simulink library "LibDBC_SCU_ch1"  (R2024b)
settings: Solver=VariableStepAuto  StartTime=0.0  StopTime=10.0  RelTol=1e-3
undefined symbols (not defined in the file): bit_packing, bit_unpacking, IO_Blk_Lib_TTC500, IO_CAN_ConfigMsg, IO_CAN_ReadMsg
libraries: simulink x59, IOBlock_Library_TTC580 x32
(part 15 of 21)

== system LibDBC_SCU_ch1/mBMS_PP ==
  note: Don't change the Names of the Blocks
  IO_CAN_ConfigMsg : Subsystem  mask(IO_CAN_ConfigMsg_Code){SampleTime=-1, ttlib=IO_Blk_Lib_TTC500, ttDescription=IO_CAN_ConfigMsg, tt_iolib_version=0.19, channel=IO_CAN_CHANNEL_1, mode=IO_CAN_MSG_READ, id_format=IO_CAN_STD_FRAME, id=0x112, ac_mask=0x7FF}
      mask help: Configures a message object for the given CAN channel.
      mask init:
      | %
      mask Help: web(which('IO_CAN.h'))
      mask TypeOptions channel: IO_CAN_CHANNEL_0  | IO_CAN_CHANNEL_1 | IO_CAN_CHANNEL_2 | IO_CAN_CHANNEL_3 | IO_CAN_CHANNEL_4 | IO_CAN_CHANNEL_5 | IO_CAN_CHANNEL_6
      mask Callback channel: %
      mask TypeOptions mode: IO_CAN_MSG_READ | IO_CAN_MSG_WRITE
      mask Callback mode: %
      mask TypeOptions id_format: IO_CAN_STD_FRAME | IO_CAN_EXT_FRAME
      mask Callback id_format: %
      mask Callback id: %
      mask Callback ac_mask: %
  IO_CAN_ReadMsg : Subsystem  mask(IO_CAN_ReadMsg_Code){SampleTime=-1, ttlib=IO_Blk_Lib_TTC500, ttDescription=IO_CAN_ReadMsg, tt_iolib_version=0.19}
      mask help: Reads a message from a given message object.
      mask init:
      | %
      mask Help: web(which('IO_CAN.h'))
  Terminator{2,6..8} (4 alike) : Terminator
  Trigger_Block : Subsystem  mask(Derate Trigger){derate=10, trigger_offset=0}
      mask prompts: trigger_offset "offset for the trigger"
      mask help: derate "n": every n-th cylce a trigger is submitted
  bit_unpacking1 : Subsystem  LoadFcn=|  mask(bit_unpacking_Code){SampleTime=-1, ttlib=IO_Blk_Lib_TTC500, ttDescription=bit_unpacking, tt_iolib_version=0.26, Endianness=little, Format=unsigned, Inversion=off, Startbit=0, Width_bits=16, Factor=0.1, Offset=0}
      | try
      | %
      | %Upgrade Information - standard BEGIN
      | new_color = 'blue';
      | new_ver = '0.26';
      | act_ver = get_param(gcb,'tt_iolib_version');
      | if not(strcmp(act_ver,new_ver))
      |     disp(['Upgrade block: ',gcb,char(10),'       Version: ',act_ver,' to ',new_ver]);
      |     %switch - case for specific upgrade information e.g. additional parameter required 
      |     %Change appearance and version information
      |     set_param(gcb,'ForegroundColor',new_color);
      |     set_param(gcb,'tt_iolib_version',new_ver);
      | end
      | %Upgrade Information - standard END
      | catch
      | %Standard catch section BEGIN
      | errordlg('An error occurred in a callback of the TTC580-BlockLib. Please open the Diagnostic Viewer for further details');
      | disp(' ');
      | disp('------------------------------------------------------------');
      | disp('An error occurred in a callback of the TTC580-BlockLib.');
      | disp(['Please check the parameters in the mask of ',gcb]);
      | disp('If you do not encounter any violations, then please '); 
      | disp('copy the following lines and report this to support@ttcontrol.com ');
      | disp('<< begin of error message dump >>');
      | disp(['Version of TTC580-BlockLib: ', get_param(gcb,'tt_iolib_version')]);
      | disp(get_param(gcb,'ttDescription'));
      | disp(gcb);
      | x=lasterror;disp(x.message);
      | disp(get_param(gcb,'MaskValues'));
      | disp(version);
      | disp(computer);
      | disp('<< end of error message dump >>');
      | disp('------------------------------------------------------------');
      | disp(' ');
      | %Standard catch section END
      | end
      mask help:
      | Block to read in CAN signal from a specified position within 64bit field.
      | For "Factor" and "Offset" the definition of Vector's CANdb applies:
      | [Physical value] = ( [Raw value] * [Factor] ) + [Offset]
      | with Raw value of a signal being the value as it is transmitted in the CAN-network
      | Verification capabilities are supported.
      mask init: same as LibDBC_SCU_ch1/EXT_BalancingRequest/bit_packing1
      mask Help: web([which('usermanual.html'),'#',lower(get_param(gcb,'ttDescription'))])
      mask TypeOptions Endianness: big | little
      mask Callback Endianness: %
      mask TypeOptions Format: unsigned | signed | real32
      mask Callback Format: %
      mask Callback Inversion: %
      mask Callback Startbit: %
      mask Callback Width_bits: %
      mask Callback Factor: %
      mask Callback Offset: %
  bit_unpacking2 : Subsystem  LoadFcn=|  mask(bit_unpacking_Code){SampleTime=-1, ttlib=IO_Blk_Lib_TTC500, ttDescription=bit_unpacking, tt_iolib_version=0.26, Endianness=little, Format=unsigned, Inversion=off, Startbit=16, Width_bits=16, Factor=1, Offset=0}
      | try
      | %
      | %Upgrade Information - standard BEGIN
      | new_color = 'blue';
      | new_ver = '0.26';
      | act_ver = get_param(gcb,'tt_iolib_version');
      | if not(strcmp(act_ver,new_ver))
      |     disp(['Upgrade block: ',gcb,char(10),'       Version: ',act_ver,' to ',new_ver]);
      |     %switch - case for specific upgrade information e.g. additional parameter required 
      |     %Change appearance and version information
      |     set_param(gcb,'ForegroundColor',new_color);
      |     set_param(gcb,'tt_iolib_version',new_ver);
      | end
      | %Upgrade Information - standard END
      | catch
      | %Standard catch section BEGIN
      | errordlg('An error occurred in a callback of the TTC580-BlockLib. Please open the Diagnostic Viewer for further details');
      | disp(' ');
      | disp('------------------------------------------------------------');
      | disp('An error occurred in a callback of the TTC580-BlockLib.');
      | disp(['Please check the parameters in the mask of ',gcb]);
      | disp('If you do not encounter any violations, then please '); 
      | disp('copy the following lines and report this to support@ttcontrol.com ');
      | disp('<< begin of error message dump >>');
      | disp(['Version of TTC580-BlockLib: ', get_param(gcb,'tt_iolib_version')]);
      | disp(get_param(gcb,'ttDescription'));
      | disp(gcb);
      | x=lasterror;disp(x.message);
      | disp(get_param(gcb,'MaskValues'));
      | disp(version);
      | disp(computer);
      | disp('<< end of error message dump >>');
      | disp('------------------------------------------------------------');
      | disp(' ');
      | %Standard catch section END
      | end
      mask help:
      | Block to read in CAN signal from a specified position within 64bit field.
      | For "Factor" and "Offset" the definition of Vector's CANdb applies:
      | [Physical value] = ( [Raw value] * [Factor] ) + [Offset]
      | with Raw value of a signal being the value as it is transmitted in the CAN-network
      | Verification capabilities are supported.
      mask init: same as LibDBC_SCU_ch1/EXT_BalancingRequest/bit_packing1
      mask Help: web([which('usermanual.html'),'#',lower(get_param(gcb,'ttDescription'))])
      mask TypeOptions Endianness: big | little
      mask Callback Endianness: %
      mask TypeOptions Format: unsigned | signed | real32
      mask Callback Format: %
      mask Callback Inversion: %
      mask Callback Startbit: %
      mask Callback Width_bits: %
      mask Callback Factor: %
      mask Callback Offset: %
  bit_unpacking3 : Subsystem  LoadFcn=|  mask(bit_unpacking_Code){SampleTime=-1, ttlib=IO_Blk_Lib_TTC500, ttDescription=bit_unpacking, tt_iolib_version=0.26, Endianness=little, Format=unsigned, Inversion=off, Startbit=32, Width_bits=16, Factor=0.1, Offset=0}
      | try
      | %
      | %Upgrade Information - standard BEGIN
      | new_color = 'blue';
      | new_ver = '0.26';
      | act_ver = get_param(gcb,'tt_iolib_version');
      | if not(strcmp(act_ver,new_ver))
      |     disp(['Upgrade block: ',gcb,char(10),'       Version: ',act_ver,' to ',new_ver]);
      |     %switch - case for specific upgrade information e.g. additional parameter required 
      |     %Change appearance and version information
      |     set_param(gcb,'ForegroundColor',new_color);
      |     set_param(gcb,'tt_iolib_version',new_ver);
      | end
      | %Upgrade Information - standard END
      | catch
      | %Standard catch section BEGIN
      | errordlg('An error occurred in a callback of the TTC580-BlockLib. Please open the Diagnostic Viewer for further details');
      | disp(' ');
      | disp('------------------------------------------------------------');
      | disp('An error occurred in a callback of the TTC580-BlockLib.');
      | disp(['Please check the parameters in the mask of ',gcb]);
      | disp('If you do not encounter any violations, then please '); 
      | disp('copy the following lines and report this to support@ttcontrol.com ');
      | disp('<< begin of error message dump >>');
      | disp(['Version of TTC580-BlockLib: ', get_param(gcb,'tt_iolib_version')]);
      | disp(get_param(gcb,'ttDescription'));
      | disp(gcb);
      | x=lasterror;disp(x.message);
      | disp(get_param(gcb,'MaskValues'));
      | disp(version);
      | disp(computer);
      | disp('<< end of error message dump >>');
      | disp('------------------------------------------------------------');
      | disp(' ');
      | %Standard catch section END
      | end
      mask help:
      | Block to read in CAN signal from a specified position within 64bit field.
      | For "Factor" and "Offset" the definition of Vector's CANdb applies:
      | [Physical value] = ( [Raw value] * [Factor] ) + [Offset]
      | with Raw value of a signal being the value as it is transmitted in the CAN-network
      | Verification capabilities are supported.
      mask init: same as LibDBC_SCU_ch1/EXT_BalancingRequest/bit_packing1
      mask Help: web([which('usermanual.html'),'#',lower(get_param(gcb,'ttDescription'))])
      mask TypeOptions Endianness: big | little
      mask Callback Endianness: %
      mask TypeOptions Format: unsigned | signed | real32
      mask Callback Format: %
      mask Callback Inversion: %
      mask Callback Startbit: %
      mask Callback Width_bits: %
      mask Callback Factor: %
      mask Callback Offset: %
  bit_unpacking4 : Subsystem  LoadFcn=|  mask(bit_unpacking_Code){SampleTime=-1, ttlib=IO_Blk_Lib_TTC500, ttDescription=bit_unpacking, tt_iolib_version=0.26, Endianness=little, Format=unsigned, Inversion=off, Startbit=48, Width_bits=16, Factor=1, Offset=0}
      | try
      | %
      | %Upgrade Information - standard BEGIN
      | new_color = 'blue';
      | new_ver = '0.26';
      | act_ver = get_param(gcb,'tt_iolib_version');
      | if not(strcmp(act_ver,new_ver))
      |     disp(['Upgrade block: ',gcb,char(10),'       Version: ',act_ver,' to ',new_ver]);
      |     %switch - case for specific upgrade information e.g. additional parameter required 
      |     %Change appearance and version information
      |     set_param(gcb,'ForegroundColor',new_color);
      |     set_param(gcb,'tt_iolib_version',new_ver);
      | end
      | %Upgrade Information - standard END
      | catch
      | %Standard catch section BEGIN
      | errordlg('An error occurred in a callback of the TTC580-BlockLib. Please open the Diagnostic Viewer for further details');
      | disp(' ');
      | disp('------------------------------------------------------------');
      | disp('An error occurred in a callback of the TTC580-BlockLib.');
      | disp(['Please check the parameters in the mask of ',gcb]);
      | disp('If you do not encounter any violations, then please '); 
      | disp('copy the following lines and report this to support@ttcontrol.com ');
      | disp('<< begin of error message dump >>');
      | disp(['Version of TTC580-BlockLib: ', get_param(gcb,'tt_iolib_version')]);
      | disp(get_param(gcb,'ttDescription'));
      | disp(gcb);
      | x=lasterror;disp(x.message);
      | disp(get_param(gcb,'MaskValues'));
      | disp(version);
      | disp(computer);
      | disp('<< end of error message dump >>');
      | disp('------------------------------------------------------------');
      | disp(' ');
      | %Standard catch section END
      | end
      mask help:
      | Block to read in CAN signal from a specified position within 64bit field.
      | For "Factor" and "Offset" the definition of Vector's CANdb applies:
      | [Physical value] = ( [Raw value] * [Factor] ) + [Offset]
      | with Raw value of a signal being the value as it is transmitted in the CAN-network
      | Verification capabilities are supported.
      mask init: same as LibDBC_SCU_ch1/EXT_BalancingRequest/bit_packing1
      mask Help: web([which('usermanual.html'),'#',lower(get_param(gcb,'ttDescription'))])
      mask TypeOptions Endianness: big | little
      mask Callback Endianness: %
      mask TypeOptions Format: unsigned | signed | real32
      mask Callback Format: %
      mask Callback Inversion: %
      mask Callback Startbit: %
      mask Callback Width_bits: %
      mask Callback Factor: %
      mask Callback Offset: %
  PP_I_chrg : Outport  VectorParamsAs1DForOutWhenUnconnected=off
  PP_Pwr_chrg : Outport  Port=2  VectorParamsAs1DForOutWhenUnconnected=off
  PP_I_dschrg : Outport  Port=3  VectorParamsAs1DForOutWhenUnconnected=off
  PP_Pwr_dschrg : Outport  Port=4  VectorParamsAs1DForOutWhenUnconnected=off
  ErrorCode : Outport  Port=5  VectorParamsAs1DForOutWhenUnconnected=off
  wires:
  IO_CAN_ReadMsg/3(buffer_length) -> Terminator8/1
  IO_CAN_ReadMsg/4(buffer_id_format) -> Terminator7/1
  IO_CAN_ReadMsg/5(buffer_id) -> Terminator6/1
  IO_CAN_ConfigMsg/2(handle) -> IO_CAN_ReadMsg/1(handle)
  IO_CAN_ConfigMsg/1(ErrorCode) -> Terminator2/1
  Trigger_Block/1(Trigger) -> IO_CAN_ReadMsg/Enable
  IO_CAN_ReadMsg/1(ErrorCode) -> ErrorCode/1
  IO_CAN_ReadMsg/2(buffer_data) -> bit_unpacking1/1(Data_in), bit_unpacking2/1(Data_in), bit_unpacking3/1(Data_in), bit_unpacking4/1(Data_in)
  bit_unpacking1/1(Data_out) -> PP_I_chrg/1
  bit_unpacking2/1(Data_out) -> PP_Pwr_chrg/1
  bit_unpacking3/1(Data_out) -> PP_I_dschrg/1
  bit_unpacking4/1(Data_out) -> PP_Pwr_dschrg/1

== system LibDBC_SCU_ch1/mBMS_RI_OCV_Approx ==
  note: Don't change the Names of the Blocks
  IO_CAN_ConfigMsg : Subsystem  mask(IO_CAN_ConfigMsg_Code){SampleTime=-1, ttlib=IO_Blk_Lib_TTC500, ttDescription=IO_CAN_ConfigMsg, tt_iolib_version=0.19, channel=IO_CAN_CHANNEL_1, mode=IO_CAN_MSG_READ, id_format=IO_CAN_STD_FRAME, id=0x113, ac_mask=0x7FF}
      mask help: Configures a message object for the given CAN channel.
      mask init:
      | %
      mask Help: web(which('IO_CAN.h'))
      mask TypeOptions channel: IO_CAN_CHANNEL_0  | IO_CAN_CHANNEL_1 | IO_CAN_CHANNEL_2 | IO_CAN_CHANNEL_3 | IO_CAN_CHANNEL_4 | IO_CAN_CHANNEL_5 | IO_CAN_CHANNEL_6
      mask Callback channel: %
      mask TypeOptions mode: IO_CAN_MSG_READ | IO_CAN_MSG_WRITE
      mask Callback mode: %
      mask TypeOptions id_format: IO_CAN_STD_FRAME | IO_CAN_EXT_FRAME
      mask Callback id_format: %
      mask Callback id: %
      mask Callback ac_mask: %
  IO_CAN_ReadMsg : Subsystem  mask(IO_CAN_ReadMsg_Code){SampleTime=-1, ttlib=IO_Blk_Lib_TTC500, ttDescription=IO_CAN_ReadMsg, tt_iolib_version=0.19}
      mask help: Reads a message from a given message object.
      mask init:
      | %
      mask Help: web(which('IO_CAN.h'))
  Terminator{2,6..8} (4 alike) : Terminator
  Trigger_Block : Subsystem  mask(Derate Trigger){derate=10, trigger_offset=0}
      mask prompts: trigger_offset "offset for the trigger"
      mask help: derate "n": every n-th cylce a trigger is submitted
  bit_unpacking1 : Subsystem  LoadFcn=|  mask(bit_unpacking_Code){SampleTime=-1, ttlib=IO_Blk_Lib_TTC500, ttDescription=bit_unpacking, tt_iolib_version=0.26, Endianness=little, Format=unsigned, Inversion=off, Startbit=0, Width_bits=16, Factor=0.01, Offset=0}
      | try
      | %
      | %Upgrade Information - standard BEGIN
      | new_color = 'blue';
      | new_ver = '0.26';
      | act_ver = get_param(gcb,'tt_iolib_version');
      | if not(strcmp(act_ver,new_ver))
      |     disp(['Upgrade block: ',gcb,char(10),'       Version: ',act_ver,' to ',new_ver]);
      |     %switch - case for specific upgrade information e.g. additional parameter required 
      |     %Change appearance and version information
      |     set_param(gcb,'ForegroundColor',new_color);
      |     set_param(gcb,'tt_iolib_version',new_ver);
      | end
      | %Upgrade Information - standard END
      | catch
      | %Standard catch section BEGIN
      | errordlg('An error occurred in a callback of the TTC580-BlockLib. Please open the Diagnostic Viewer for further details');
      | disp(' ');
      | disp('------------------------------------------------------------');
      | disp('An error occurred in a callback of the TTC580-BlockLib.');
      | disp(['Please check the parameters in the mask of ',gcb]);
      | disp('If you do not encounter any violations, then please '); 
      | disp('copy the following lines and report this to support@ttcontrol.com ');
      | disp('<< begin of error message dump >>');
      | disp(['Version of TTC580-BlockLib: ', get_param(gcb,'tt_iolib_version')]);
      | disp(get_param(gcb,'ttDescription'));
      | disp(gcb);
      | x=lasterror;disp(x.message);
      | disp(get_param(gcb,'MaskValues'));
      | disp(version);
      | disp(computer);
      | disp('<< end of error message dump >>');
      | disp('------------------------------------------------------------');
      | disp(' ');
      | %Standard catch section END
      | end
      mask help:
      | Block to read in CAN signal from a specified position within 64bit field.
      | For "Factor" and "Offset" the definition of Vector's CANdb applies:
      | [Physical value] = ( [Raw value] * [Factor] ) + [Offset]
      | with Raw value of a signal being the value as it is transmitted in the CAN-network
      | Verification capabilities are supported.
      mask init: same as LibDBC_SCU_ch1/EXT_BalancingRequest/bit_packing1
      mask Help: web([which('usermanual.html'),'#',lower(get_param(gcb,'ttDescription'))])
      mask TypeOptions Endianness: big | little
      mask Callback Endianness: %
      mask TypeOptions Format: unsigned | signed | real32
      mask Callback Format: %
      mask Callback Inversion: %
      mask Callback Startbit: %
      mask Callback Width_bits: %
      mask Callback Factor: %
      mask Callback Offset: %
  bit_unpacking2 : Subsystem  LoadFcn=|  mask(bit_unpacking_Code){SampleTime=-1, ttlib=IO_Blk_Lib_TTC500, ttDescription=bit_unpacking, tt_iolib_version=0.26, Endianness=little, Format=unsigned, Inversion=off, Startbit=16, Width_bits=16, Factor=0.01, Offset=0}
      | try
      | %
      | %Upgrade Information - standard BEGIN
      | new_color = 'blue';
      | new_ver = '0.26';
      | act_ver = get_param(gcb,'tt_iolib_version');
      | if not(strcmp(act_ver,new_ver))
      |     disp(['Upgrade block: ',gcb,char(10),'       Version: ',act_ver,' to ',new_ver]);
      |     %switch - case for specific upgrade information e.g. additional parameter required 
      |     %Change appearance and version information
      |     set_param(gcb,'ForegroundColor',new_color);
      |     set_param(gcb,'tt_iolib_version',new_ver);
      | end
      | %Upgrade Information - standard END
      | catch
      | %Standard catch section BEGIN
      | errordlg('An error occurred in a callback of the TTC580-BlockLib. Please open the Diagnostic Viewer for further details');
      | disp(' ');
      | disp('------------------------------------------------------------');
      | disp('An error occurred in a callback of the TTC580-BlockLib.');
      | disp(['Please check the parameters in the mask of ',gcb]);
      | disp('If you do not encounter any violations, then please '); 
      | disp('copy the following lines and report this to support@ttcontrol.com ');
      | disp('<< begin of error message dump >>');
      | disp(['Version of TTC580-BlockLib: ', get_param(gcb,'tt_iolib_version')]);
      | disp(get_param(gcb,'ttDescription'));
      | disp(gcb);
      | x=lasterror;disp(x.message);
      | disp(get_param(gcb,'MaskValues'));
      | disp(version);
      | disp(computer);
      | disp('<< end of error message dump >>');
      | disp('------------------------------------------------------------');
      | disp(' ');
      | %Standard catch section END
      | end
      mask help:
      | Block to read in CAN signal from a specified position within 64bit field.
      | For "Factor" and "Offset" the definition of Vector's CANdb applies:
      | [Physical value] = ( [Raw value] * [Factor] ) + [Offset]
      | with Raw value of a signal being the value as it is transmitted in the CAN-network
      | Verification capabilities are supported.
      mask init: same as LibDBC_SCU_ch1/EXT_BalancingRequest/bit_packing1
      mask Help: web([which('usermanual.html'),'#',lower(get_param(gcb,'ttDescription'))])
      mask TypeOptions Endianness: big | little
      mask Callback Endianness: %
      mask TypeOptions Format: unsigned | signed | real32
      mask Callback Format: %
      mask Callback Inversion: %
      mask Callback Startbit: %
      mask Callback Width_bits: %
      mask Callback Factor: %
      mask Callback Offset: %
  bit_unpacking3 : Subsystem  LoadFcn=|  mask(bit_unpacking_Code){SampleTime=-1, ttlib=IO_Blk_Lib_TTC500, ttDescription=bit_unpacking, tt_iolib_version=0.26, Endianness=little, Format=unsigned, Inversion=off, Startbit=32, Width_bits=16, Factor=0.01, Offset=0}
      | try
      | %
      | %Upgrade Information - standard BEGIN
      | new_color = 'blue';
      | new_ver = '0.26';
      | act_ver = get_param(gcb,'tt_iolib_version');
      | if not(strcmp(act_ver,new_ver))
      |     disp(['Upgrade block: ',gcb,char(10),'       Version: ',act_ver,' to ',new_ver]);
      |     %switch - case for specific upgrade information e.g. additional parameter required 
      |     %Change appearance and version information
      |     set_param(gcb,'ForegroundColor',new_color);
      |     set_param(gcb,'tt_iolib_version',new_ver);
      | end
      | %Upgrade Information - standard END
      | catch
      | %Standard catch section BEGIN
      | errordlg('An error occurred in a callback of the TTC580-BlockLib. Please open the Diagnostic Viewer for further details');
      | disp(' ');
      | disp('------------------------------------------------------------');
      | disp('An error occurred in a callback of the TTC580-BlockLib.');
      | disp(['Please check the parameters in the mask of ',gcb]);
      | disp('If you do not encounter any violations, then please '); 
      | disp('copy the following lines and report this to support@ttcontrol.com ');
      | disp('<< begin of error message dump >>');
      | disp(['Version of TTC580-BlockLib: ', get_param(gcb,'tt_iolib_version')]);
      | disp(get_param(gcb,'ttDescription'));
      | disp(gcb);
      | x=lasterror;disp(x.message);
      | disp(get_param(gcb,'MaskValues'));
      | disp(version);
      | disp(computer);
      | disp('<< end of error message dump >>');
      | disp('------------------------------------------------------------');
      | disp(' ');
      | %Standard catch section END
      | end
      mask help:
      | Block to read in CAN signal from a specified position within 64bit field.
      | For "Factor" and "Offset" the definition of Vector's CANdb applies:
      | [Physical value] = ( [Raw value] * [Factor] ) + [Offset]
      | with Raw value of a signal being the value as it is transmitted in the CAN-network
      | Verification capabilities are supported.
      mask init: same as LibDBC_SCU_ch1/EXT_BalancingRequest/bit_packing1
      mask Help: web([which('usermanual.html'),'#',lower(get_param(gcb,'ttDescription'))])
      mask TypeOptions Endianness: big | little
      mask Callback Endianness: %
      mask TypeOptions Format: unsigned | signed | real32
      mask Callback Format: %
      mask Callback Inversion: %
      mask Callback Startbit: %
      mask Callback Width_bits: %
      mask Callback Factor: %
      mask Callback Offset: %
  bit_unpacking4 : Subsystem  LoadFcn=|  mask(bit_unpacking_Code){SampleTime=-1, ttlib=IO_Blk_Lib_TTC500, ttDescription=bit_unpacking, tt_iolib_version=0.26, Endianness=little, Format=unsigned, Inversion=off, Startbit=48, Width_bits=16, Factor=0.01, Offset=0}
      | try
      | %
      | %Upgrade Information - standard BEGIN
      | new_color = 'blue';
      | new_ver = '0.26';
      | act_ver = get_param(gcb,'tt_iolib_version');
      | if not(strcmp(act_ver,new_ver))
      |     disp(['Upgrade block: ',gcb,char(10),'       Version: ',act_ver,' to ',new_ver]);
      |     %switch - case for specific upgrade information e.g. additional parameter required 
      |     %Change appearance and version information
      |     set_param(gcb,'ForegroundColor',new_color);
      |     set_param(gcb,'tt_iolib_version',new_ver);
      | end
      | %Upgrade Information - standard END
      | catch
      | %Standard catch section BEGIN
      | errordlg('An error occurred in a callback of the TTC580-BlockLib. Please open the Diagnostic Viewer for further details');
      | disp(' ');
      | disp('------------------------------------------------------------');
      | disp('An error occurred in a callback of the TTC580-BlockLib.');
      | disp(['Please check the parameters in the mask of ',gcb]);
      | disp('If you do not encounter any violations, then please '); 
      | disp('copy the following lines and report this to support@ttcontrol.com ');
      | disp('<< begin of error message dump >>');
      | disp(['Version of TTC580-BlockLib: ', get_param(gcb,'tt_iolib_version')]);
      | disp(get_param(gcb,'ttDescription'));
      | disp(gcb);
      | x=lasterror;disp(x.message);
      | disp(get_param(gcb,'MaskValues'));
      | disp(version);
      | disp(computer);
      | disp('<< end of error message dump >>');
      | disp('------------------------------------------------------------');
      | disp(' ');
      | %Standard catch section END
      | end
      mask help:
      | Block to read in CAN signal from a specified position within 64bit field.
      | For "Factor" and "Offset" the definition of Vector's CANdb applies:
      | [Physical value] = ( [Raw value] * [Factor] ) + [Offset]
      | with Raw value of a signal being the value as it is transmitted in the CAN-network
      | Verification capabilities are supported.
      mask init: same as LibDBC_SCU_ch1/EXT_BalancingRequest/bit_packing1
      mask Help: web([which('usermanual.html'),'#',lower(get_param(gcb,'ttDescription'))])
      mask TypeOptions Endianness: big | little
      mask Callback Endianness: %
      mask TypeOptions Format: unsigned | signed | real32
      mask Callback Format: %
      mask Callback Inversion: %
      mask Callback Startbit: %
      mask Callback Width_bits: %
      mask Callback Factor: %
      mask Callback Offset: %
  Cell_Ri_Ch_OCV : Outport  VectorParamsAs1DForOutWhenUnconnected=off
  Cell_Ri_DCh_OCV : Outport  Port=2  VectorParamsAs1DForOutWhenUnconnected=off
  Cell_Ri_Ch_Approx : Outport  Port=3  VectorParamsAs1DForOutWhenUnconnected=off
  Cell_Ri_DCh_Approx : Outport  Port=4  VectorParamsAs1DForOutWhenUnconnected=off
  ErrorCode : Outport  Port=5  VectorParamsAs1DForOutWhenUnconnected=off
  wires:
  IO_CAN_ReadMsg/3(buffer_length) -> Terminator8/1
  IO_CAN_ReadMsg/4(buffer_id_format) -> Terminator7/1
  IO_CAN_ReadMsg/5(buffer_id) -> Terminator6/1
  IO_CAN_ConfigMsg/2(handle) -> IO_CAN_ReadMsg/1(handle)
  IO_CAN_ConfigMsg/1(ErrorCode) -> Terminator2/1
  Trigger_Block/1(Trigger) -> IO_CAN_ReadMsg/Enable
  IO_CAN_ReadMsg/1(ErrorCode) -> ErrorCode/1
  IO_CAN_ReadMsg/2(buffer_data) -> bit_unpacking1/1(Data_in), bit_unpacking2/1(Data_in), bit_unpacking3/1(Data_in), bit_unpacking4/1(Data_in)
  bit_unpacking1/1(Data_out) -> Cell_Ri_Ch_OCV/1
  bit_unpacking2/1(Data_out) -> Cell_Ri_DCh_OCV/1
  bit_unpacking3/1(Data_out) -> Cell_Ri_Ch_Approx/1
  bit_unpacking4/1(Data_out) -> Cell_Ri_DCh_Approx/1
